simulink model "single_vertical_joint_dynamics"  (R2020b)
settings: Solver=FixedStepAuto  StartTime=0.0  StopTime=20  FixedStep=1e-3  RelTol=1e-3
settings Model: Creator=a302  LastModifiedBy=a302

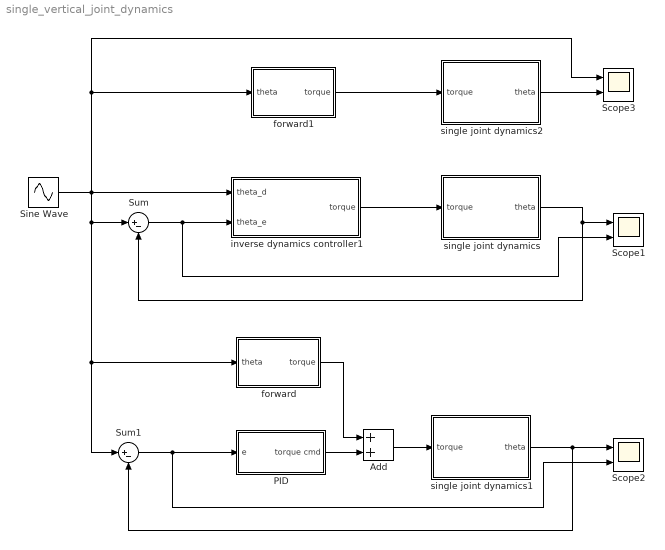
== system single_vertical_joint_dynamics ==
  Add : Sum
  PID : Subsystem  mask{Kp=50, Ki=0, Kd=10}
  Scope1 : Scope  NumInputPorts=2
  Scope2 : Scope  NumInputPorts=2
  Scope3 : Scope  NumInputPorts=2
  Sine Wave : Sin  Amplitude=-pi/2  Bias=pi/2  Phase=pi/2  SampleTime=0
  Sum : Sum  Inputs=|+-
  Sum1 : Sum  Inputs=|+-
  forward : Subsystem  mask{J=0.6, m=2, r=0.08, b=0.12, g=9.81}
  forward1 : Subsystem  mask{J=0.5, m=1, r=0.1, b=0.1, g=9.81}
  inverse dynamics controller1 : Subsystem  mask{J=0.6, m=2, r=0.08, b=0.12, g=9.81, Kp=50, Ki=0, Kd=10}
  single joint dynamics : Subsystem  mask{J=0.5, m=1, r=0.1, b=0.1, g=9.81}
      mask DialogControl DescTextVar Prompt: single joint dynamics
      mask Display: image('$imagefile'); % Use "Edit Image" on toolstrip to change.
  single joint dynamics1 : Subsystem  mask{J=0.5, m=1, r=0.1, b=0.1, g=9.81}
      mask DialogControl DescTextVar Prompt: single joint dynamics
      mask Display: image('$imagefile'); % Use "Edit Image" on toolstrip to change.
  single joint dynamics2 : Subsystem  mask{J=0.5, m=1, r=0.1, b=0.1, g=9.81}
      mask DialogControl DescTextVar Prompt: single joint dynamics
      mask Display: image('$imagefile'); % Use "Edit Image" on toolstrip to change.
  wires:
  single joint dynamics/1(theta) -> Scope1/1, Sum/2
  Sum/1 -> inverse dynamics controller1/2(theta_e), Scope1/2
  inverse dynamics controller1/1(torque) -> single joint dynamics/1(torque)
  single joint dynamics1/1(theta) -> Sum1/2, Scope2/1
  PID/1(torque cmd) -> Add/2
  Sine Wave/1 -> Scope3/1, forward1/1(theta), forward/1(theta), Sum1/1, Sum/1, inverse dynamics controller1/1(theta_d)
  Sum1/1 -> PID/1(e), Scope2/2
  Add/1 -> single joint dynamics1/1(torque)
  forward/1(torque) -> Add/1
  forward1/1(torque) -> single joint dynamics2/1(torque)
  single joint dynamics2/1(theta) -> Scope3/2

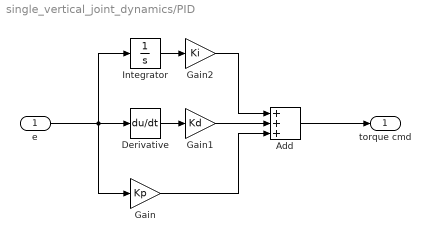
== system single_vertical_joint_dynamics/PID ==
  e : Inport
  Add : Sum  Inputs=+++
  Derivative : Derivative
  Gain : Gain  Gain=Kp
  Gain1 : Gain  Gain=Kd
  Gain2 : Gain  Gain=Ki
  Integrator : Integrator
  torque cmd : Outport
  wires:
  Gain2/1 -> Add/1
  Gain1/1 -> Add/2
  Add/1 -> torque cmd/1
  Derivative/1 -> Gain1/1
  e/1 -> Gain/1, Derivative/1, Integrator/1
  Integrator/1 -> Gain2/1
  Gain/1 -> Add/3

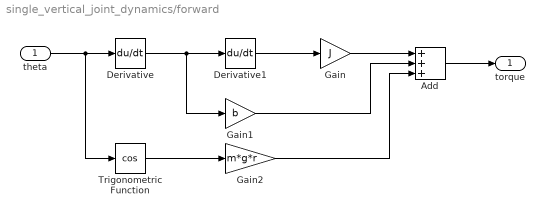
== system single_vertical_joint_dynamics/forward ==
  theta : Inport
  Add : Sum  Inputs=+++
  Derivative : Derivative
  Derivative1 : Derivative
  Gain : Gain  Gain=J
  Gain1 : Gain  Gain=b
  Gain2 : Gain  Gain=m*g*r
  Trigonometric Function : Trigonometry  Operator=cos
  torque : Outport
  wires:
  theta/1 -> Trigonometric Function/1, Derivative/1
  Trigonometric Function/1 -> Gain2/1
  Add/1 -> torque/1
  Gain2/1 -> Add/3
  Derivative/1 -> Gain1/1, Derivative1/1
  Gain1/1 -> Add/2
  Gain/1 -> Add/1
  Derivative1/1 -> Gain/1

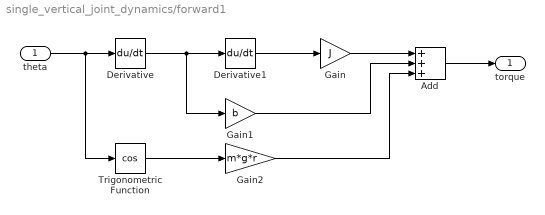
== system single_vertical_joint_dynamics/forward1 ==
  theta : Inport
  Add : Sum  Inputs=+++
  Derivative : Derivative
  Derivative1 : Derivative
  Gain : Gain  Gain=J
  Gain1 : Gain  Gain=b
  Gain2 : Gain  Gain=m*g*r
  Trigonometric Function : Trigonometry  Operator=cos
  torque : Outport
  wires:
  theta/1 -> Trigonometric Function/1, Derivative/1
  Trigonometric Function/1 -> Gain2/1
  Add/1 -> torque/1
  Gain2/1 -> Add/3
  Derivative/1 -> Gain1/1, Derivative1/1
  Gain1/1 -> Add/2
  Gain/1 -> Add/1
  Derivative1/1 -> Gain/1

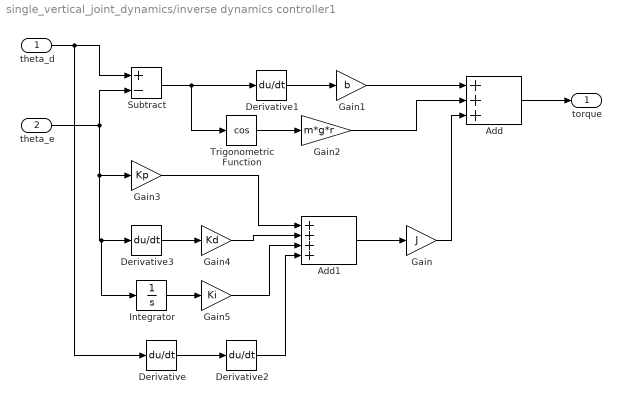
== system single_vertical_joint_dynamics/inverse dynamics controller1 ==
  theta_d : Inport
  theta_e : Inport  Port=2
  Add : Sum  Inputs=+++
  Add1 : Sum  Inputs=++++
  Derivative{,1..3} (4 alike) : Derivative
  Gain : Gain  Gain=J
  Gain1 : Gain  Gain=b
  Gain2 : Gain  Gain=m*g*r
  Gain3 : Gain  Gain=Kp
  Gain4 : Gain  Gain=Kd
  Gain5 : Gain  Gain=Ki
  Integrator : Integrator
  Subtract : Sum  Inputs=+-
  Trigonometric Function : Trigonometry  Operator=cos
  torque : Outport
  wires:
  theta_d/1 -> Subtract/1, Derivative/1
  theta_e/1 -> Integrator/1, Derivative3/1, Gain3/1, Subtract/2
  Subtract/1 -> Trigonometric Function/1, Derivative1/1
  Derivative1/1 -> Gain1/1
  Gain1/1 -> Add/1
  Gain2/1 -> Add/2
  Derivative/1 -> Derivative2/1
  Derivative3/1 -> Gain4/1
  Integrator/1 -> Gain5/1
  Gain3/1 -> Add1/1
  Gain4/1 -> Add1/2
  Gain5/1 -> Add1/3
  Derivative2/1 -> Add1/4
  Add1/1 -> Gain/1
  Gain/1 -> Add/3
  Trigonometric Function/1 -> Gain2/1
  Add/1 -> torque/1

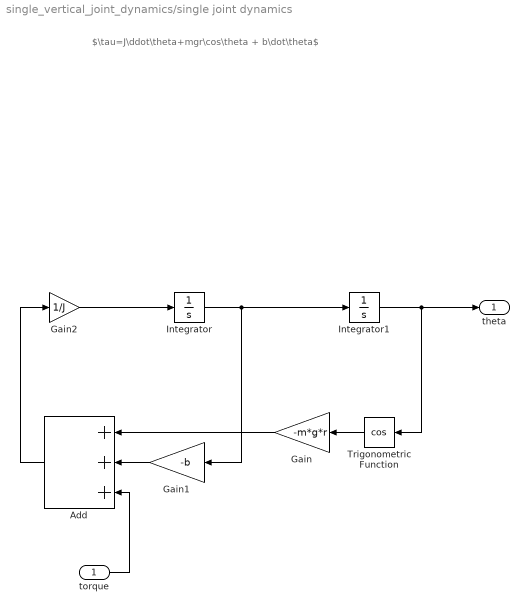
== system single_vertical_joint_dynamics/single joint dynamics ==
  note: $\tau=J\ddot\theta+mgr\cos\theta + b\dot\theta$
  torque : Inport
  Add : Sum  Inputs=+++
  Gain : Gain  Gain=-m*g*r
  Gain1 : Gain  Gain=-b
  Gain2 : Gain  Gain=1/J
  Integrator : Integrator
  Integrator1 : Integrator
  Trigonometric Function : Trigonometry  Operator=cos
  theta : Outport
  wires:
  Gain/1 -> Add/1
  Integrator/1 -> Integrator1/1, Gain1/1
  Gain2/1 -> Integrator/1
  Trigonometric Function/1 -> Gain/1
  Integrator1/1 -> theta/1, Trigonometric Function/1
  Gain1/1 -> Add/2
  Add/1 -> Gain2/1
  torque/1 -> Add/3

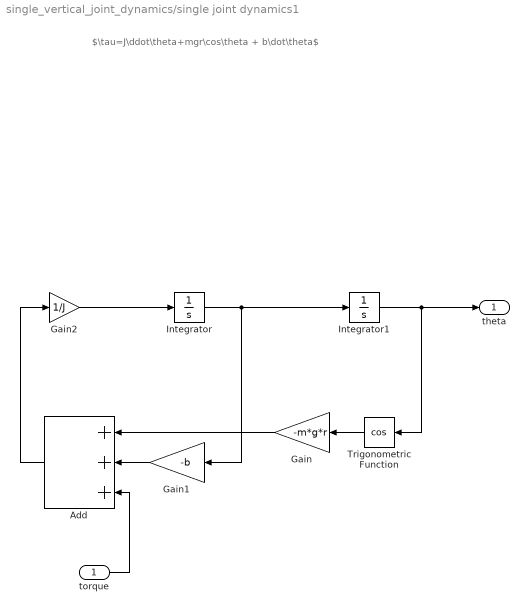
== system single_vertical_joint_dynamics/single joint dynamics1 ==
  note: $\tau=J\ddot\theta+mgr\cos\theta + b\dot\theta$
  torque : Inport
  Add : Sum  Inputs=+++
  Gain : Gain  Gain=-m*g*r
  Gain1 : Gain  Gain=-b
  Gain2 : Gain  Gain=1/J
  Integrator : Integrator
  Integrator1 : Integrator
  Trigonometric Function : Trigonometry  Operator=cos
  theta : Outport
  wires:
  Gain/1 -> Add/1
  Integrator/1 -> Integrator1/1, Gain1/1
  Gain2/1 -> Integrator/1
  Trigonometric Function/1 -> Gain/1
  Integrator1/1 -> theta/1, Trigonometric Function/1
  Gain1/1 -> Add/2
  Add/1 -> Gain2/1
  torque/1 -> Add/3

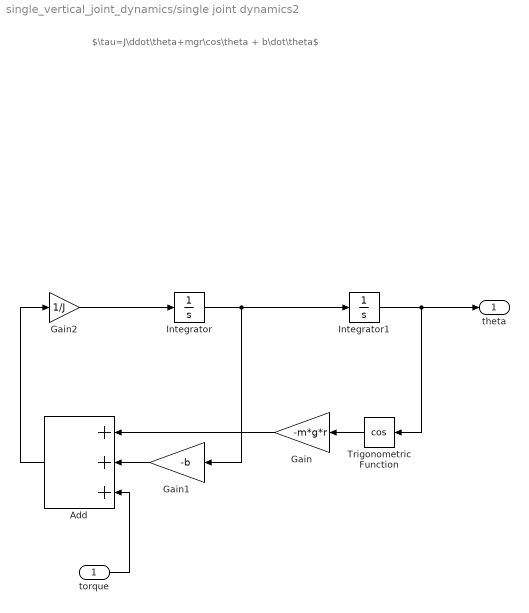
== system single_vertical_joint_dynamics/single joint dynamics2 ==
  note: $\tau=J\ddot\theta+mgr\cos\theta + b\dot\theta$
  torque : Inport
  Add : Sum  Inputs=+++
  Gain : Gain  Gain=-m*g*r
  Gain1 : Gain  Gain=-b
  Gain2 : Gain  Gain=1/J
  Integrator : Integrator
  Integrator1 : Integrator
  Trigonometric Function : Trigonometry  Operator=cos
  theta : Outport
  wires:
  Gain/1 -> Add/1
  Integrator/1 -> Integrator1/1, Gain1/1
  Gain2/1 -> Integrator/1
  Trigonometric Function/1 -> Gain/1
  Integrator1/1 -> theta/1, Trigonometric Function/1
  Gain1/1 -> Add/2
  Add/1 -> Gain2/1
  torque/1 -> Add/3
